simulink model "schemeJm2"  (R2014a)
settings: Solver=ode45  StartTime=0.0  StopTime=0.4  MaxStep=0.001  MinStep=0.0001  RelTol=1e-3
settings Model: Creator=User  LastModifiedBy=Анастасия

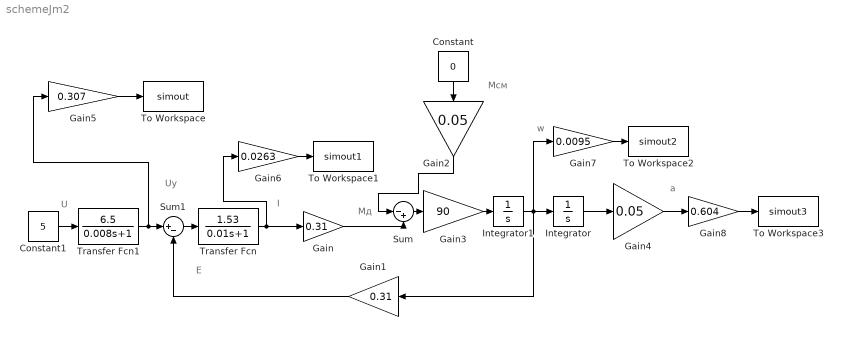
== system schemeJm2 ==
  note: E
  note: a
  note: w
  note: Мд
  note: Mсм
  note: I
  note: Uy
  note: U
  Constant : Constant  Value=0
  Constant1 : Constant  Value=5
  Gain : Gain  Gain=0.31
  Gain1 : Gain  Gain=0.31
  Gain2 : Gain  Gain=0.05
  Gain3 : Gain  Gain=90
  Gain4 : Gain  Gain=0.05
  Gain5 : Gain  Gain=0.307
  Gain6 : Gain  Gain=0.0263
  Gain7 : Gain  Gain=0.0095
  Gain8 : Gain  Gain=0.604
  Integrator : Integrator
  Integrator1 : Integrator
  Sum : Sum  Inputs=|-+
  Sum1 : Sum  Inputs=|+-
  To Workspace : ToWorkspace  VariableName=simout  SaveFormat=Timeseries  SampleTime=-1
  To Workspace1 : ToWorkspace  VariableName=simout1  SaveFormat=Timeseries  SampleTime=-1
  To Workspace2 : ToWorkspace  VariableName=simout2  SaveFormat=Timeseries  SampleTime=-1
  To Workspace3 : ToWorkspace  VariableName=simout3  SaveFormat=Timeseries  SampleTime=-1
  Transfer Fcn : TransferFcn  Numerator=[1.53]  Denominator=[0.01 1]
  Transfer Fcn1 : TransferFcn  Numerator=[6.5]  Denominator=[0.008 1]
  wires:
  Constant1/1 -> Transfer Fcn1/1
  Transfer Fcn1/1 -> Gain5/1, Sum1/1
  Transfer Fcn/1 -> Gain6/1, Gain/1
  Gain/1 -> Sum/2
  Constant/1 -> Gain2/1
  Gain2/1 -> Sum/1
  Sum/1 -> Gain3/1
  Gain3/1 -> Integrator1/1
  Integrator1/1 -> Gain7/1, Gain1/1, Integrator/1
  Gain1/1 -> Sum1/2
  Sum1/1 -> Transfer Fcn/1
  Integrator/1 -> Gain4/1
  Gain4/1 -> Gain8/1
  Gain8/1 -> To Workspace3/1
  Gain7/1 -> To Workspace2/1
  Gain6/1 -> To Workspace1/1
  Gain5/1 -> To Workspace/1
